simulink model "kinematics_model"  (R2025b)
settings: Solver=VariableStepAuto  StartTime=0.0  StopTime=10.0  RelTol=1e-3
libraries: sharedutil x1
settings Model: Creator=mahausmani  LastModifiedBy=mahausmani

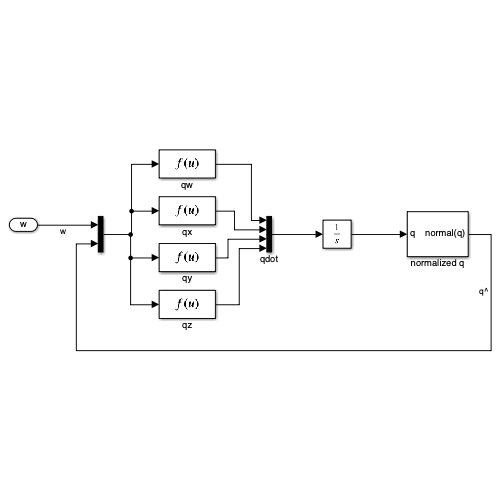
[thumbnail: Simulink's stored preview of the top-level diagram]
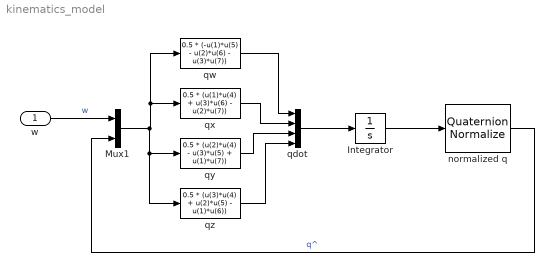
== system kinematics_model ==
  w : Inport
  Integrator : Integrator
  Mux1 : Mux  Inputs=2
  normalized q : sharedutil/Quaternion Normalize  aMode=aMode
  qdot : Mux
  qw : Fcn  Expr=0.5 * (-u(1)*u(5) - u(2)*u(6) - u(3)*u(7))
  qx : Fcn  Expr=0.5 * (u(1)*u(4) + u(3)*u(6) - u(2)*u(7))
  qy : Fcn  Expr=0.5 * (u(2)*u(4) - u(3)*u(5) + u(1)*u(7))
  qz : Fcn  Expr=0.5 * (u(3)*u(4) + u(2)*u(5) - u(1)*u(6))
  wires:
  Integrator/1 -> normalized q/1
  qdot/1 -> Integrator/1
  qz/1 -> qdot/4
  qy/1 -> qdot/3
  qx/1 -> qdot/2
  qw/1 -> qdot/1
  Mux1/1 -> qz/1, qy/1, qx/1, qw/1
  normalized q/1 -> Mux1/2  "q^"
  w/1 -> Mux1/1  "w"
